simulink model "Lung-Mechanics-Simulation-using-Lumped-Parameter-Model"  (R2023b)
settings: Solver=VariableStepAuto  StartTime=0.0  StopTime=10.0  RelTol=1e-3
settings Model: Creator=R.Dipti  LastModifiedBy=R.Dipti

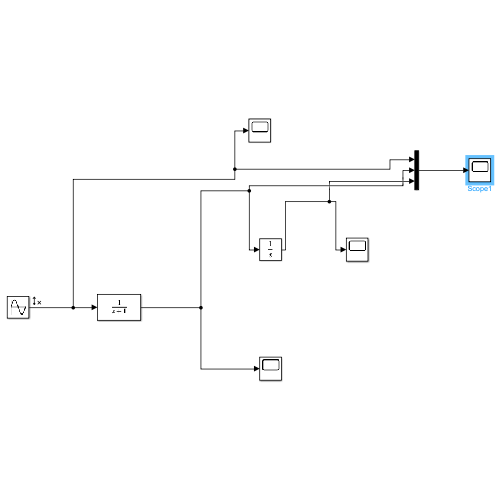
[thumbnail: Simulink's stored preview of the top-level diagram]
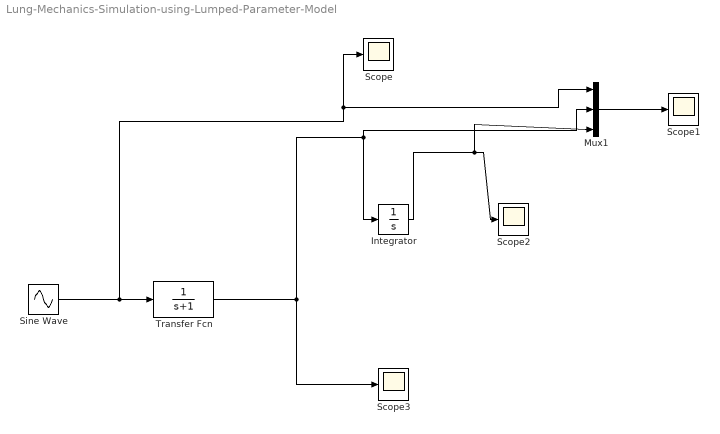
== system Lung-Mechanics-Simulation-using-Lumped-Parameter-Model ==
  Integrator : Integrator
  Mux1 : Mux  Inputs=3
  Scope{,1..3} (4 alike) : Scope
  Sine Wave : Sin  SampleTime=0
  Transfer Fcn : TransferFcn  Denominator=[1 1]
  wires:
  Sine Wave/1 -> Mux1/1, Scope/1, Transfer Fcn/1
  Integrator/1 -> Mux1/3, Scope2/1
  Transfer Fcn/1 -> Scope3/1, Mux1/2, Integrator/1
  Mux1/1 -> Scope1/1
